simulink model "AUAV_V3_TestSensors_"  (R2015a)
settings: Solver=FixedStepDiscrete  StartTime=0.0  StopTime=10.0  FixedStep=T  RelTol=1e-3
PreLoadFcn:
  | %T = 0.0025;
  | MavlinkBus;
  | mcuInit;
  | % Baro Altitude Computation
  | % =========================
  | basePressure = 98192.64;
  | baseTemp = 288.215;
  | lapseRate = -0.00198122;
  | baseHeight = 0;
values from neighbouring files (symbols this model uses):
  apSampleTime = 0.01    [mcuInit.m]
  latlong_WP = 1    [mcuInit.m]
  mavlink_attitude_t = Simulink.Bus    [MavlinkBusMarcello.m]
  mavlink_gps_raw_int_t = Simulink.Bus    [MavlinkBus.m]    (also in MavlinkBusMarcello.m)
  mavlink_raw_imu_t = Simulink.Bus    [MavlinkBus.m]    (also in MavlinkBusMarcello.m)
  mavlink_scaled_pressure_t = Simulink.Bus    [MavlinkBus.m]    (also in MavlinkBusMarcello.m)
  mavlink_servo_output_raw_t = Simulink.Bus    [MavlinkBusMarcello.m]
  mavlink_sys_status_t = Simulink.Bus    [MavlinkBus.m]    (also in MavlinkBusMarcello.m)
  T = 0.01    [mcuInit.m]
  Xpoints = [0 0]    [mcuInit.m]
  Ypoints = [0 0]    [mcuInit.m]
  Zpoints = [0 0]    [mcuInit.m]
undefined symbols (not defined in the file or in its folder): A0, A14, A15, A2, A3, A4, A5, A6, accBiasRateLimit, B0, bankCommandLimit, barAdjust, baroCutoff, baroCutTemp, cubeAccelGain16405, cubeGyroGain16405, cubeMagGain16405, D0, D11, D7, D8, daLimit, data, daTrimMax, daTrimMin, deLimit, deTrimMax, deTrimMin, drLimit, drTrimMax, drTrimMin, dtLimit, dtTrimMax, dtTrimMin, F2, F3, G0, G13, G15, gaind, GS_location, gyroBiasRateLimit, IC1max, IPStar, ISA_g, Max, maxAcc, MaxDwnPthStar, maxDynPressure, maxEta, mlParamInterface, ms, OC1max, P112, P125, P127, P16, P20, P21, P30 ... (+26)
undefined symbols (not defined in the file): baroOffset, baroScale, barTGain1, barTGain2, barTMean1, barTMean2, bda, bde, bdr, bdt, bICda, bICde, bICdr, bICdt, derivativesConstant, lowRateSensorCutoff, mainSensorCutoff, mda, mde, mdr, mdt, mICda, mICde, mICdr, mICdt, pitotOffset, pitotScale, pitTGain1, pitTGain2, pitTMean1, pitTMean2, powerOffset, powerScale, pressureSensorCutoff, tempOffset, tempScale, vzCutoff, xCutoff, yCutoff
libraries: MCHP_Blockset x150, simulink x84, SLUGS_Library x31, aerolibconvert2 x6, aerolibutil x4, aerolibtransform2 x3, dspmtrx3 x2, aerolibobsolete x2
(part 10 of 20)

== system AUAV_V3_TestSensors_/Sensor_Data_Adapter/Sensor Suite ==
  HIL_flag : Inport
  Raw HIL : Inport  Port=2
  " GPS is Ublox" : Subsystem
  "ADIS16405 Signal Cond " : Subsystem
  Compute CPU Load : Subsystem
  Data Type Conversion{4..7} (4 alike) : DataTypeConversion  OutDataTypeStr=single
  Demux : Demux
  Demux1 : Demux
  Goto4 : Goto  Commented=on  GotoTag=IntDiag
  Goto5 : Goto  Commented=on  GotoTag=charDiag
  If no HIL then Read all the Sensors : Subsystem
  If no HIL then update Air Data : Subsystem
  Logical Operator : Logic  Operator=NOT  AllPortsSameDT=off  OutDataTypeStr=boolean
  Low Pass Filtering,Temperature Compensation and Calibration : Subsystem
  Sensor DSC Diag [updateSensorMcuState.c]1 : MCHP_Blockset/User Functions/C Function Call  ParseFilesChkbx=off  ListFunctions1=Custom Function  Function1=extern void updateSensorDiag(real32_T* u1);  AddHeaderDeclaration=off  Function1Type=when block is updated (default)  Fct1BlockIn=u1[4]  FctReturnBlockOut=off  DataCollected=0  ORDERING=None  SampleTime=.01  MCHP_MASTERLINK=|  PinDigitalInput=[]  PinDigitalOutput=[]  PinAnalogInput=[]
      | AUAV_V3_TestSensors_/Microchip Master
      | AUAV V3 Board
      | Busy Flag on D2 (RA6)
  Switch : Switch  Criteria=u2 ~= 0  SampleTime=0.01
  Switch1 : Switch  Criteria=u2 ~= 0  SampleTime=0.01
  Update the Load and Power Data [updateSensorMcuState.c]1 : MCHP_Blockset/User Functions/C Function Call  ParseFilesChkbx=off  ListFunctions1=Custom Function  Function1=extern void updateLoadData(uint8_T u1, uint16_T u2);  AddHeaderDeclaration=off  Function1Type=when block is updated (default)  FctReturnBlockOut=off  DataCollected=0  ORDERING=None  SampleTime=.01  MCHP_MASTERLINK=|  PinDigitalInput=[]  PinDigitalOutput=[]  PinAnalogInput=[]
      | AUAV_V3_TestSensors_/Microchip Master
      | AUAV V3 Board
      | Busy Flag on D2 (RA6)
  myMux Fun : MATLAB Function  TreatAsAtomicUnit=on
  myMux Fun1 : MATLAB Function  TreatAsAtomicUnit=on
  Omega (rad/s) : Outport
  Accel (m/s^2) : Outport  Port=2
  Mag (mG) : Outport  Port=3
  Baro Alt (m) : Outport  Port=4
  GPS : Outport  Port=5
  wires:
  If no HIL then Read all the Sensors/1(Sensors) -> Switch/3
  Logical Operator/1 -> If no HIL then Read all the Sensors/Enable, [Not_HIL]
  Demux/1 -> "ADIS16405 Signal Cond "/1(Gyro Raw)  "Gyro"
  Demux1/1 -> Low Pass Filtering,Temperature Compensation and Calibration/1(Baro raw)
  Demux1/2 -> Low Pass Filtering,Temperature Compensation and Calibration/2(Pitot raw)
  Demux1/4 -> Low Pass Filtering,Temperature Compensation and Calibration/4(Therm Raw)
  Demux/3 -> "ADIS16405 Signal Cond "/3(Mag Raw)  "Mag"
  Demux1/3 -> Low Pass Filtering,Temperature Compensation and Calibration/3(Power Raw)
  Low Pass Filtering,Temperature Compensation and Calibration/2(Pitot (Pa)) -> myMux Fun/1(u1), [Float1Diag]
  Low Pass Filtering,Temperature Compensation and Calibration/3(Static (Pa)) -> myMux Fun/2(u2)
  myMux Fun/1(y) -> If no HIL then update Air Data/1(AirData)
  Low Pass Filtering,Temperature Compensation and Calibration/4(Temp (0.1 C)) -> myMux Fun/3(u3)
  Compute CPU Load/1(Load (%)) -> Update the Load and Power Data [updateSensorMcuState.c]1/1
  Low Pass Filtering,Temperature Compensation and Calibration/5(Power (V)) -> Update the Load and Power Data [updateSensorMcuState.c]1/2
  Demux/2 -> "ADIS16405 Signal Cond "/2(Accel Raw)  "Accel"
  myMux Fun1/1(y) -> Sensor DSC Diag [updateSensorMcuState.c]1/1
  Data Type Conversion5/1 -> myMux Fun1/1(u1)  "float"
  Data Type Conversion4/1 -> myMux Fun1/2(u2)  "float"
  Data Type Conversion6/1 -> myMux Fun1/3(u3)  "int"
  Data Type Conversion7/1 -> myMux Fun1/4(u4)  "char"
  [Float1Diag] -> Data Type Conversion5/1
  [Float2Diag] -> Data Type Conversion4/1
  [IntDiag] -> Data Type Conversion6/1
  [charDiag] -> Data Type Conversion7/1
  [Not_HIL] -> If no HIL then update Air Data/Enable
  If no HIL then update Air Data/1(Out1) -> [Float2Diag]
  "ADIS16405 Signal Cond "/1(Omega (rad/s)) -> Omega (rad/s)/1
  "ADIS16405 Signal Cond "/2(Accel (m/s^2)) -> Accel (m/s^2)/1
  "ADIS16405 Signal Cond "/3(Mags (mG)) -> Mag (mG)/1
  Raw HIL/1 -> Switch/1
  HIL_flag/1 -> [HIL], Switch/2, Logical Operator/1
  Switch/1 -> Demux/1
  Low Pass Filtering,Temperature Compensation and Calibration/1(Baro Alt (m)) -> Baro Alt (m)/1
  Demux/4 -> Demux1/1
  [Not_HIL] -> Switch1/2
  Switch1/1 -> GPS/1
  " GPS is Ublox"/1(GPS Main) -> Switch1/3
  If no HIL then Read all the Sensors/2(GPS) -> Switch1/1

== system AUAV_V3_TestSensors_/Servo In Out/Convert to Microseconds ==
  PWM : Inport
  Convert to Microseconds : Gain  Gain=0.4
  Data Type Conversion : DataTypeConversion  OutDataTypeStr=uint16
  uS : Outport
  wires:
  Data Type Conversion/1 -> uS/1
  PWM/1 -> Convert to Microseconds/1
  Convert to Microseconds/1 -> Data Type Conversion/1

== system AUAV_V3_TestSensors_/Servo In Out/Convert to Microseconds1 ==
  PWM : Inport
  Convert to Microseconds : Gain  Gain=0.4
  Data Type Conversion : DataTypeConversion  OutDataTypeStr=uint16
  uS : Outport
  wires:
  Data Type Conversion/1 -> uS/1
  PWM/1 -> Convert to Microseconds/1
  Convert to Microseconds/1 -> Data Type Conversion/1

== system AUAV_V3_TestSensors_/Servo In Out/Convert to Microseconds2 ==
  PWM : Inport
  Convert to Microseconds : Gain  Gain=0.4
  Data Type Conversion : DataTypeConversion  OutDataTypeStr=uint16
  uS : Outport
  wires:
  Data Type Conversion/1 -> uS/1
  PWM/1 -> Convert to Microseconds/1
  Convert to Microseconds/1 -> Data Type Conversion/1

== system AUAV_V3_TestSensors_/Servo In Out/Mixing ==
  note: Pitch positif : go down
      | Yaw positive : turn left
  Pitch : Inport
  Roll : Inport  Port=2
  Sum : Sum  Inputs=-+  SaturateOnIntegerOverflow=on  OutDataTypeStr=Inherit: Same as first input
  Sum1 : Sum  SaturateOnIntegerOverflow=on  OutDataTypeStr=Inherit: Same as first input
  Cmd Servo Left : Outport
  Cmd Servo Right : Outport  Port=2
  wires:
  Pitch/1 -> Sum1/1, Sum/1
  Roll/1 -> Sum/2, Sum1/2
  Sum/1 -> Cmd Servo Left/1
  Sum1/1 -> Cmd Servo Right/1

== system AUAV_V3_TestSensors_/Trim Vals [updated 4.28.16]/Bufffer IC ==
  Pilot Console : Inport
  Buffer IC Channel : MATLAB Function  TreatAsAtomicUnit=on
  Buffer IC Channel1 : MATLAB Function  TreatAsAtomicUnit=on
  Buffer IC Channel2 : MATLAB Function  TreatAsAtomicUnit=on
  Buffer IC Channel3 : MATLAB Function  TreatAsAtomicUnit=on
  Demux : Demux
  dT_buf : Outport
  dA_buf : Outport  Port=2
  dR_buf : Outport  Port=3
  dE_buf : Outport  Port=4
  wires:
  Demux/1 -> Buffer IC Channel/1(latest)
  Demux/2 -> Buffer IC Channel1/1(latest)
  Demux/3 -> Buffer IC Channel2/1(latest)
  Demux/4 -> Buffer IC Channel3/1(latest)
  Pilot Console/1 -> Demux/1
  Buffer IC Channel/1(history) -> dT_buf/1
  Buffer IC Channel1/1(history) -> dA_buf/1
  Buffer IC Channel2/1(history) -> dR_buf/1
  Buffer IC Channel3/1(history) -> dE_buf/1

== system AUAV_V3_TestSensors_/Trim Vals [updated 4.28.16]/Control Surface Input ==
  2 sec  tau : Subsystem  mask(Tustin1stOrderLowpassAutoInitialCondition){f=0.1, T=T}
      mask prompts: f "Lowpass Frequency"; T "Sample Time"
      mask help: Takes a 3db rolloff frequency (in Hz, NOT radians/s) and a sample time. Performs a symbolic Tustin conversion and implements in a discrete filter. The initial output of the filter is set by the first sample.
      mask Help: Enter the desired 3db rolloff frequency in Hz and the sample time. Initial conditions are sampled automatically.
      mask Display: fprintf('%.2f Hz lowpass',f)
  2 sec  tau1 : Subsystem  mask(Tustin1stOrderLowpassAutoInitialCondition){f=0.1, T=T}
      mask prompts: f "Lowpass Frequency"; T "Sample Time"
      mask help: Takes a 3db rolloff frequency (in Hz, NOT radians/s) and a sample time. Performs a symbolic Tustin conversion and implements in a discrete filter. The initial output of the filter is set by the first sample.
      mask Help: Enter the desired 3db rolloff frequency in Hz and the sample time. Initial conditions are sampled automatically.
      mask Display: fprintf('%.2f Hz lowpass',f)
  Data Type Conversion1 : DataTypeConversion  OutDataTypeStr=uint16
  Data Type Conversion2 : DataTypeConversion  OutDataTypeStr=single
  Data Type Conversion3 : DataTypeConversion  OutDataTypeStr=single
  Data Type Conversion4 : DataTypeConversion  OutDataTypeStr=uint16
  Input Capture : MCHP_Blockset/Pulse Input//Output/Input Capture  IntPriority=6  Channel="[1     2     3     4     5     6     7     8]"  Channel_OLD="[1  2  3  4  5  6  7  8]"  PIN_IC1=Dynamic Options  PIN_IC1_TXT=D0 / P64 / Pin[72]  PIN_IC2=Dynamic Options  PIN_IC2_TXT=D8 / P72 / Pin[68]  PIN_IC3=Dynamic Options  PIN_IC3_TXT=D11 / P75 / Pin[71]  PIN_IC4=Dynamic Options  PIN_IC4_TXT=A15 / P31 / Pin[67]  PIN_IC5=Dynamic Options  PIN_IC5_TXT=A5 / P21 / Pin[61]  PIN_IC6=Dynamic Options  PIN_IC6_TXT=A14 / P30 / Pin[66]  PIN_IC7=Dynamic Options  PIN_IC7_TXT=A4 / P20 / Pin[60]  PIN_IC8=Dynamic Options  PIN_IC8_TXT=A0 / P16 / Pin[17]  PIN_IC9=Dynamic Options  PIN_IC9_TXT=A0 / P16 / Pin[17]  PIN_IC10=Dynamic Options  PIN_IC10_TXT=A0 / P16 / Pin[17]  PIN_IC11=Dynamic Options  PIN_IC11_TXT=A0 / P16 / Pin[17]  PIN_IC12=Dynamic Options  PIN_IC12_TXT=A0 / P16 / Pin[17]  PIN_IC13=Dynamic Options  PIN_IC13_TXT=A0 / P16 / Pin[17]  PIN_IC14=Dynamic Options  PIN_IC14_TXT=A0 / P16 / Pin[17]  PIN_IC15=Dynamic Options  PIN_IC15_TXT=A0 / P16 / Pin[17]  PIN_IC16=Dynamic Options  PIN_IC16_TXT=A0 / P16 / Pin[17]  Channel_UP_Down_Periode="[1     1     1     1     1     1     1     1]"  MaxChannel="[0.003   0.003   0.003   0.003   0.003   0.003   0.003   0.003]"  SafeMarge="[0     0     0     0     0     0     0     0]"  MaxChannelValue="2.^[ 14.680  14.680  14.680  14.680  14.680  14.680  14.680  14.680]  =>  [26249  26249  26249  26249  26249  26249  26249  26249]"  ICxmax="[26249  26249  26249  26249  26249  26249  26249  26249]"  Timer="[1  1  1  1  1  1  1  1]"  ChangeDetected="[0     0     0     0     0     0     0     0]"  ChangeDetectedPortRef=3  SampleTime=.01  Status=OK  MCHP_PORT={Input Capture 1}{IC1}6:0:P64;{Input Capture 2}{IC2}6:0:P72;{Input Capture 3}{IC3}6:0:P75;{Input Capture 4}{IC4}6:0:P31;{Input Capture 5}{IC5}6:0:P21;{Input Capture 6}{IC6}6:0:P30;{Input Capture 7}{IC7}6:0:P20;{Input Capture 8}{IC8}6:0:P16;  MCHP_TIMER_REQUEST="{Input Capture 1}{IC1}6:0:1:0:[1  2  3  4  5]:210000;{Input Capture 1}{IC1}6:0:1:0:[1  2  3  4  5]:210000;{Input Capture 1}{IC1}6:0:1:0:[1  2  3  4  5]:210000;{Input Capture 1}{IC1}6:0:1:0:[1  2  3  4  5]:210000;{Input Capture 1}{IC1}6:0:1:0:[1  2  3  4  5]:210000;{Input Capture 1}{IC1}6:0:1:0:[1  2  3  4  5]:210000;{Input Capture 1}{IC1}6:0:1:0:[1  2  3  4  5]:210000;{Input Capture 1}{IC1}6:0:1:0:[1  2  3  4  5]:210000;"  MCHP_TIMER_RESULT=[1 26249.000000000011 ;1 26249.000000000011 ;1 26249.000000000011 ;1 26249.000000000011 ;1 26249.000000000011 ;1 26249.000000000011 ;1 26249.000000000011 ;1 26249.000000000011 ]  MCHP_MASTERLINK=|
      | AUAV_V3_TestSensors/Microchip Master
      | AUAV V3 Board
      | Busy Flag on D2 (RA6)
  Update Control Surface DATA : DataStoreWrite  DialogController=Simulink.DDGSource  DataStoreName=mlPilotConsoleData  DataStoreElements=mlPilotConsoleData.chan1_raw#mlPilotConsoleData.chan2_raw#mlPilotConsoleData.chan3_raw#mlPilotConsoleData.chan4_raw#mlPilotConsoleData.chan5_raw#mlPilotConsoleData.chan6_raw#mlPilotConsoleData.chan7_raw#mlPilotConsoleData.chan8_raw
  myMux Fun1 : MATLAB Function  TreatAsAtomicUnit=on
  myMux Fun5 : MATLAB Function  TreatAsAtomicUnit=on
  Pilot Console : Outport
  Voltage/Current Sensor : Outport  Port=2
  wires:
  Input Capture/7 -> Data Type Conversion3/1, Update Control Surface DATA/7
  myMux Fun1/1(y) -> Voltage/Current Sensor/1
  Input Capture/6 -> Update Control Surface DATA/6, Data Type Conversion2/1
  2 sec  tau/1(Out1) -> Data Type Conversion1/1
  2 sec  tau1/1(Out1) -> Data Type Conversion4/1
  Data Type Conversion1/1 -> myMux Fun1/1(u1)
  Data Type Conversion4/1 -> myMux Fun1/2(u2)
  Data Type Conversion2/1 -> 2 sec  tau/1(In1)
  Data Type Conversion3/1 -> 2 sec  tau1/1(In1)
  Input Capture/1 -> myMux Fun5/1(u1), Update Control Surface DATA/1
  Input Capture/4 -> myMux Fun5/4(u4), Update Control Surface DATA/4
  Input Capture/5 -> myMux Fun5/5(u5), Update Control Surface DATA/5
  Input Capture/2 -> myMux Fun5/2(u2), Update Control Surface DATA/2
  Input Capture/3 -> myMux Fun5/3(u3), Update Control Surface DATA/3
  myMux Fun5/1(y) -> Pilot Console/1
  Input Capture/8 -> Update Control Surface DATA/8

== system AUAV_V3_TestSensors_/Trim Vals [updated 4.28.16]/Convert to Microseconds  ==
  IC : Inport
  Convert to Microseconds : Gain  Gain=0.2
  Data Type Conversion : DataTypeConversion  OutDataTypeStr=uint16
  uS : Outport
  wires:
  Convert to Microseconds/1 -> Data Type Conversion/1
  IC/1 -> Convert to Microseconds/1
  Data Type Conversion/1 -> uS/1

== system AUAV_V3_TestSensors_/Trim Vals [updated 4.28.16]/Detect Transition High to Low ==
  Switch : Inport
  IC1 : InitialCondition  Value=0
  Logical Operator : Logic  Operator=NOT  AllPortsSameDT=off  OutDataTypeStr=boolean
  Subsystem : Subsystem
  Transition : Outport
  wires:
  Switch/1 -> Logical Operator/1
  IC1/1 -> Subsystem/1(WP Fly)
  Logical Operator/1 -> IC1/1
  Subsystem/1(Just Enab) -> Transition/1

== system AUAV_V3_TestSensors_/Trim Vals [updated 4.28.16]/Grab I.C. ==
  dT_buf : Inport
  dA_buf : Inport  Port=2
  dR_buf : Inport  Port=3
  dE_buf : Inport  Port=4
  Enable : EnablePort
  2 : MCHP_Blockset/User Functions/C Function Call  ParseFilesChkbx=off  ListFunctions1=Custom Function  Function1=extern uint16_T meanFilter5(uint16_T* u1);  AddHeaderDeclaration=off  Function1Type=when block is updated (default)  FctReturnBlockOut=on  Fct1BlockOut=y1  DataCollected=0  ORDERING=None  SampleTime=-1  MCHP_MASTERLINK=|  PinDigitalInput=[]  PinDigitalOutput=[]  PinAnalogInput=[]
      | AUAV_V3_TestSensors_/Microchip Master
      | AUAV V3 Board
      | Busy Flag on D2 (RA6)
  3 : MCHP_Blockset/User Functions/C Function Call  ParseFilesChkbx=off  ListFunctions1=Custom Function  Function1=extern uint16_T meanFilter5(uint16_T* u1);  AddHeaderDeclaration=off  Function1Type=when block is updated (default)  FctReturnBlockOut=on  Fct1BlockOut=y1  DataCollected=0  ORDERING=None  SampleTime=-1  MCHP_MASTERLINK=|  PinDigitalInput=[]  PinDigitalOutput=[]  PinAnalogInput=[]
      | AUAV_V3_TestSensors_/Microchip Master
      | AUAV V3 Board
      | Busy Flag on D2 (RA6)
  4 : MCHP_Blockset/User Functions/C Function Call  ParseFilesChkbx=off  ListFunctions1=Custom Function  Function1=extern uint16_T meanFilter5(uint16_T* u1);  AddHeaderDeclaration=off  Function1Type=when block is updated (default)  FctReturnBlockOut=on  Fct1BlockOut=y1  DataCollected=0  ORDERING=None  SampleTime=-1  MCHP_MASTERLINK=|  PinDigitalInput=[]  PinDigitalOutput=[]  PinAnalogInput=[]
      | AUAV_V3_TestSensors_/Microchip Master
      | AUAV V3 Board
      | Busy Flag on D2 (RA6)
  Choose the Median navSupport.c [updated 4.28.16] : MCHP_Blockset/User Functions/C Function Call  ParseFilesChkbx=off  ListFunctions1=Custom Function  Function1=extern uint16_T meanFilter5(uint16_T* u1);  AddHeaderDeclaration=off  Function1Type=when block is updated (default)  FctReturnBlockOut=on  Fct1BlockOut=y1  DataCollected=0  ORDERING=None  SampleTime=-1  MCHP_MASTERLINK=|  PinDigitalInput=[]  PinDigitalOutput=[]  PinAnalogInput=[]
      | AUAV_V3_TestSensors_/Microchip Master
      | AUAV V3 Board
      | Busy Flag on D2 (RA6)
  "Convert to Microseconds " : Subsystem
  Convert to Microseconds 1 : Subsystem
  Convert to Microseconds 2 : Subsystem
  Convert to Microseconds 3 : Subsystem
  Convert to Rad : Subsystem  mask{slopem=mICdt, interceptb=bICdt}
      mask prompts: slopem "Slope"; interceptb "Intercept"
  Convert to Rad1 : Subsystem  mask{slopem=mICda, interceptb=bICda}
      mask prompts: slopem "Slope"; interceptb "Intercept"
  Convert to Rad2 : Subsystem  mask{slopem=mICdr, interceptb=bICdr}
      mask prompts: slopem "Slope"; interceptb "Intercept"
  Convert to Rad3 : Subsystem  mask{slopem=mICde, interceptb=bICde}
      mask prompts: slopem "Slope"; interceptb "Intercept"
  "[-2  2] deg" : Saturate  UpperLimit=daTrimMax  LowerLimit=daTrimMin
  "[-2  2] deg " : Saturate  UpperLimit=drTrimMax  LowerLimit=drTrimMin
  "[-2  2] deg  " : Saturate  UpperLimit=deTrimMax  LowerLimit=deTrimMin
  "[0.55 0.68]" : Saturate  UpperLimit=dtTrimMax  LowerLimit=dtTrimMin
  dA : Constant  OutDataTypeStr=uint8
  dE : Constant  Value=3  OutDataTypeStr=uint8
  dR : Constant  Value=2  OutDataTypeStr=uint8
  dT : Constant  Value=0  OutDataTypeStr=uint8
  update dA Trim updateControlMcu.c : MCHP_Blockset/User Functions/C Function Call  ParseFilesChkbx=off  ListFunctions1=Custom Function  Function1=extern void updatePWMTrim(uint16_T* u1, uint8_T* u2);  AddHeaderDeclaration=off  Function1Type=when block is updated (default)  FctReturnBlockOut=on  DataCollected=0  ORDERING=None  SampleTime=-1  MCHP_MASTERLINK=|  PinDigitalInput=[]  PinDigitalOutput=[]  PinAnalogInput=[]
      | AUAV_V3_TestSensors_/Microchip Master
      | AUAV V3 Board
      | Busy Flag on D2 (RA6)
  update dE Trim updateControlMcu.c : MCHP_Blockset/User Functions/C Function Call  ParseFilesChkbx=off  ListFunctions1=Custom Function  Function1=extern void updatePWMTrim(uint16_T* u1, uint8_T* u2);  AddHeaderDeclaration=off  Function1Type=when block is updated (default)  FctReturnBlockOut=on  DataCollected=0  ORDERING=None  SampleTime=-1  MCHP_MASTERLINK=|  PinDigitalInput=[]  PinDigitalOutput=[]  PinAnalogInput=[]
      | AUAV_V3_TestSensors_/Microchip Master
      | AUAV V3 Board
      | Busy Flag on D2 (RA6)
  update dR Trim updateControlMcu.c : MCHP_Blockset/User Functions/C Function Call  ParseFilesChkbx=off  ListFunctions1=Custom Function  Function1=extern void updatePWMTrim(uint16_T* u1, uint8_T* u2);  AddHeaderDeclaration=off  Function1Type=when block is updated (default)  FctReturnBlockOut=on  DataCollected=0  ORDERING=None  SampleTime=-1  MCHP_MASTERLINK=|  PinDigitalInput=[]  PinDigitalOutput=[]  PinAnalogInput=[]
      | AUAV_V3_TestSensors_/Microchip Master
      | AUAV V3 Board
      | Busy Flag on D2 (RA6)
  update dT Trim updateControlMcu.c [updated 4.28.16] : MCHP_Blockset/User Functions/C Function Call  ParseFilesChkbx=off  ListFunctions1=Custom Function  Function1=extern void updatePWMTrim(uint16_T* u1, uint8_T* u2);  AddHeaderDeclaration=off  Function1Type=when block is updated (default)  FctReturnBlockOut=on  DataCollected=0  ORDERING=None  SampleTime=-1  MCHP_MASTERLINK=|  PinDigitalInput=[]  PinDigitalOutput=[]  PinAnalogInput=[]
      | AUAV_V3_TestSensors_/Microchip Master
      | AUAV V3 Board
      | Busy Flag on D2 (RA6)
  dT_trim (abs) : Outport
  dA_trim (rad) : Outport  Port=2
  dR_trim (rad) : Outport  Port=3
  dE_trim (rad) : Outport  Port=4
  wires:
  Convert to Rad/1(Angle (rad)) -> dT_trim (abs)/1
  Convert to Rad2/1(Angle (rad)) -> dR_trim (rad)/1
  Convert to Rad3/1(Angle (rad)) -> dE_trim (rad)/1
  Choose the Median navSupport.c [updated 4.28.16]/1 -> "[0.55 0.68]"/1
  2/1 -> "[-2  2] deg"/1
  3/1 -> "[-2  2] deg "/1
  4/1 -> "[-2  2] deg  "/1
  dT_buf/1 -> Choose the Median navSupport.c [updated 4.28.16]/1
  dA_buf/1 -> 2/1
  dR_buf/1 -> 3/1
  dR/1 -> update dR Trim updateControlMcu.c/2
  dE/1 -> update dE Trim updateControlMcu.c/2
  dT/1 -> update dT Trim updateControlMcu.c [updated 4.28.16]/2
  dA/1 -> update dA Trim updateControlMcu.c/2
  "[0.55 0.68]"/1 -> Convert to Rad/1(IC), "Convert to Microseconds "/1(IC)
  "[-2  2] deg"/1 -> Convert to Rad1/1(IC), Convert to Microseconds 1/1(IC)
  "[-2  2] deg "/1 -> Convert to Rad2/1(IC), Convert to Microseconds 2/1(IC)
  "[-2  2] deg  "/1 -> Convert to Rad3/1(IC), Convert to Microseconds 3/1(IC)
  Convert to Rad1/1(Angle (rad)) -> dA_trim (rad)/1
  "Convert to Microseconds "/1(uS) -> update dT Trim updateControlMcu.c [updated 4.28.16]/1
  Convert to Microseconds 1/1(uS) -> update dA Trim updateControlMcu.c/1
  Convert to Microseconds 2/1(uS) -> update dR Trim updateControlMcu.c/1
  Convert to Microseconds 3/1(uS) -> update dE Trim updateControlMcu.c/1
  dE_buf/1 -> 4/1

== system AUAV_V3_TestSensors_/Trim Vals [updated 4.28.16]/Mean Filter the Transition ==
  Failsafe : Inport
  Buffer Failsafe Channel : MATLAB Function  TreatAsAtomicUnit=on
  Choose the Median [navSupport.c] [updated 5.1.16] : MCHP_Blockset/User Functions/C Function Call  ParseFilesChkbx=off  ListFunctions1=Custom Function  Function1=extern uint16_T meanFilter5(uint8_T *u1);  AddHeaderDeclaration=on  Function1Type=when block is updated (default)  Fct1BlockIn=u1  FctReturnBlockOut=on  DataCollected=0  ORDERING=None  SampleTime=-1  MCHP_MASTERLINK=|  PinDigitalInput=[]  PinDigitalOutput=[]  PinAnalogInput=[]
      | AUAV_V3_TestSensors_/Microchip Master
      | AUAV V3 Board
      | Busy Flag on D2 (RA6)
  Data Type Conversion : DataTypeConversion  OutDataTypeStr=uint16
  Data Type Conversion1 : DataTypeConversion  OutDataTypeStr=uint8
  filtered : Outport
  wires:
  Choose the Median [navSupport.c] [updated 5.1.16]/1 -> filtered/1
  Data Type Conversion/1 -> Buffer Failsafe Channel/1(latest)
  Failsafe/1 -> Data Type Conversion/1
  Data Type Conversion1/1 -> Choose the Median [navSupport.c] [updated 5.1.16]/1
  Buffer Failsafe Channel/1(history) -> Data Type Conversion1/1

== system AUAV_V3_TestSensors_/Update PWM Commands and Send Telemetry [updated 4.27.16]/Convert to Microseconds ==
  PWM : Inport
  Convert to Microseconds : Gain  Gain=0.2
  Data Type Conversion : DataTypeConversion  OutDataTypeStr=uint16
  uS : Outport
  wires:
  Data Type Conversion/1 -> uS/1
  PWM/1 -> Convert to Microseconds/1
  Convert to Microseconds/1 -> Data Type Conversion/1

== system AUAV_V3_TestSensors_/Update PWM Commands and Send Telemetry [updated 4.27.16]/Generate PWM Signals Based on the Control Type ==
  note: Navigation Modes:
      | 2 -> PT
      | 3 -> Waypoint
      | 4 -> Mid Level
      | 8-> Sel PT
      | 9-> ISR
      | 10 -> Line Patrol
  PWM(rad) : Inport
  Pilot Console (IC) : Inport  Port=2
  isManual? : Inport  Port=3
  Nav Mode : Inport  Port=4
  Data Type Conversion : DataTypeConversion  OutDataTypeStr=uint16
  Data Type Conversion1 : DataTypeConversion  OutDataTypeStr=uint8
  If : If  NumInputs=2  IfExpression=u2 == 1  ElseIfExpressions=((u1 == 3) | (u1 == 4) | (u1 == 9) | (u1 == 10)), u1 == 2, u1 == 8  ShowElse=off  SampleTime=.01
  If  Control Type Is Manual : Subsystem  TreatAsAtomicUnit=on
  If  Control Type Is Passthrough : Subsystem  TreatAsAtomicUnit=on
  If  Control Type Is Selective Passthrough : Subsystem  TreatAsAtomicUnit=on
  "If  Control Type Is Wp, ISR, LP or  Mid Lvl Cmds" : Subsystem  TreatAsAtomicUnit=on
  Merge : Merge  Inputs=4
  PWM : Outport
  wires:
  If/1 -> If  Control Type Is Manual/Action
  If/2 -> "If  Control Type Is Wp, ISR, LP or  Mid Lvl Cmds"/Action
  If/3 -> If  Control Type Is Passthrough/Action
  If/4 -> If  Control Type Is Selective Passthrough/Action
  If  Control Type Is Manual/1(PWM) -> Merge/1
  "If  Control Type Is Wp, ISR, LP or  Mid Lvl Cmds"/1(PWM (abs)) -> Merge/2
  If  Control Type Is Passthrough/1(PWM (abs)) -> Merge/3
  If  Control Type Is Selective Passthrough/1(PWM) -> Merge/4
  PWM(rad)/1 -> "If  Control Type Is Wp, ISR, LP or  Mid Lvl Cmds"/1(PWM(rad)), If  Control Type Is Selective Passthrough/1(PWM(rad))
  Pilot Console (IC)/1 -> If  Control Type Is Manual/1(Pilot (IC)), If  Control Type Is Passthrough/1(Pilot (IC)), If  Control Type Is Selective Passthrough/2(Pilot (IC))
  Merge/1 -> Data Type Conversion/1
  Data Type Conversion/1 -> PWM/1
  isManual?/1 -> If/2
  Nav Mode/1 -> Data Type Conversion1/1
  Data Type Conversion1/1 -> If/1

== system AUAV_V3_TestSensors_/Update PWM Commands and Send Telemetry [updated 4.27.16]/Send_Cmd_HIL ==
  Enable : EnablePort
  COMP_ID : Constant  OutDataTypeStr=uint8
  Get Raw Commands : DataStoreRead  DialogController=Simulink.DDGSource  DataStoreName=mlPwmCommands  DataStoreElements=mlPwmCommands
  Get time5 : DataStoreRead  DataStoreName=time_since_boot_usec  DataStoreElements=time_since_boot_usec
  PackRawServo : MCHP_Blockset/User Functions/C Function Call  ParseFilesChkbx=on  ListFunctions1=Custom Function  Function1=uint16_t HIL_PackRawServo(uint8_t system_id, uint8_t component_id, mavlink_servo_output_raw_t mlPwmCommands ,uint32_t time_usec)  AddHeaderDeclaration=on  Function1Type=when block is updated (default)  Fct1BlockIn="system_id  , component_id  , mlPwmCommands  , time_usec"  FctReturnBlockOut=on  DataCollected="s.chksm=reshape({ '638503-Feb-2015 20:58:10','251913-Sep-2016 12:15:14','1628414-Sep-2016 10:06:29','3754120-Sep-2016 10:12:03','360317-Jun-2016 15:34:16','7114620-Sep-2016 10:38:54','954931-Aug-2016 15:03:40','295520-Sep-2016 10:30:42','268124-Jun-2016 00:23:34','556017-Jun-2016 15:34:16','963217-Jun-2016 15:34:16','1086024-Jun-2016 00:23:34','372414-Sep-2016 14:01:55','998814-Sep-2016 11:55:45','509015-Sep-2016 09:12:19'},1,15);s.File1=reshape({ '  void  newCircBuffer(CBRef cB)','  void  freeCircBuffer(CBRef* cB)','  void  freeCircBuffer(CBRef* cB)',' unsigned int  getLength(CBRef cB)','  int  readHead(CBRef cB)','  int  readTail(CBRef cB)',' unsigned char  peak(CBRef cB)',' unsigned char  readFront(CBRef cB)',' unsigned char  writeBack(CBRef cB, unsigned char data)','  void  makeEmpty(CBRef cB)','  void  printCircBuf(CBRef cB)'},1,11);s.File2=reshape({ '  void  uartBufferInit(void)','  void  __attribute__((__interrupt__, no_auto_psv)) _U4RXInterrupt(void)','  void  getGPSRawData(unsigned char* gpsBuffer)',' unsigned char  isGPSNovatel(void)'},1,4);s.File3=reshape({ '  char  hex2char(char halfhex)','  float  degMinToDeg(unsigned char degrees, float minutes)',' unsigned char  gpsUbloxSeparate(unsigned char* outStream)','  void  gpsUbloxParse(void)','  void  getGpsUbloxMainData(float* data)','  char  gpSmbl(char symbl)',' unsigned char  myTokenizer(char* stringToTokenize, char token, char * returnToken)','  void  parseRMC(unsigned char* stream)','  void  parseGGA(unsigned char* stream)',' unsigned char  getChecksum(unsigned char* sentence, unsigned char size)','  void  gpsDebugMsg(unsigned char buf)'},1,11);s.File4=reshape({ '  void  uartMavlinkBufferInit(void)','  void __attribute__((__interrupt__,__auto_psv__)) _U1RXInterrupt(void)','  uint8_t  isFinite(float s)','  void  InitParameterInterface(void)','  void  protDecodeMavlink(void)','  uint16_t  MissionInterfaceResponse(uint8_t system_id, uint8_t component_id)','  uint16_t  ParameterInterfaceResponse(uint8_t system_id, uint8_t component_id)','  uint16_t  PackHeartBeat(uint8_t system_id, uint8_t component_id)','  uint16_t  PackTextMsg(uint8_t system_id, uint8_t component_id, unsigned char buf)','  uint16_t  PackRawIMU(uint8_t system_id, uint8_t component_id, mavlink_raw_imu_t mlRawIMUData ,uint32_t time_usec)','  uint16_t  PackGpsRawInt(uint8_t system_id, uint8_t component_id, mavlink_gps_raw_int_t mlRawGpsDataInt ,uint32_t time_usec)','  uint16_t  PackScaledPressure(uint8_t system_id, uint8_t component_id, mavlink_scaled_pressure_t mlAirData ,uint32_t time_usec)','  uint16_t  PackSysStatus(uint8_t system_id, uint8_t component_id, mavlink_sys_status_t mlSysStatus)','  uint16_t  PackRawServo(uint8_t system_id, uint8_t component_id, mavlink_servo_output_raw_t mlPwmCommands ,uint32_t time_usec)','  uint16_t  HIL_PackRawServo(uint8_t system_id, uint8_t component_id, mavlink_servo_output_raw_t mlPwmCommands ,uint32_t time_usec)','  uint16_t  PackRawRC(uint8_t system_id, uint8_t component_id, mavlink_rc_channels_raw_t mlRC_Commands ,uint32_t time_usec)','  uint16_t  PackVFR_HUD(uint8_t system_id, uint8_t component_id, mavlink_vfr_hud_t mlVfr_hud ,uint32_t time_usec)','  char  sendQGCDebugMessage(const char * dbgMessage, char severity, unsigned char* bytesToAdd, char positionStart)','  void  TxN_Data_OverU1(uint16_t N)','  void  TxN_Data_OverU4(uint16_t N)'},1,20);s.File5=reshape({ '  float  myAtan2(float num, float denom)','  float  myPow(float x, float toTheN)','  float  mySqrt(float x)','  float  myAbs(float x)','  float  myAtan(float x)','  float  myAsin(float x)','  float  mySin(float x)','  float  myCos(float x)','  float  myTan(float x)','  float  myAcos(float x)','  float  myExp(float x)','  void  hugeDelay(void)','  void  smallDelay(void)','  void  tinyDelay(void)','  void  printToUart2(const char *fmt, ...)'},1,15);s.File6=reshape({ '  void  sendTelemetryMavlink(unsigned char* dataOut)','  void  uart2Init(void)','  void  gsRead(unsigned char* gsChunk)','  void  prepareTelemetryMavlink(unsigned char* dataOut)','  void  prepareTelemetryMavlink(unsigned char* dataOut)','  void  sendTelemetryMavlink(unsigned char* dataOut)','  void  copyBufferToDMA1(unsigned char size)','  void  send2GS(unsigned char* protData)','  uint8_t  clearWaypointsFrom(uint8_t startingWp)','  void  addMessageToSpiOut(mavlink_message_t* msg)'},1,10);s.File7={ '  void  populateParameterInterface(void)'};s.File8={ '  void  mavlinkInit(void)'};s.File9=reshape({ '  void  updatePWM(unsigned short * PWMData)','  void  updatePWMTrim(unsigned short PWMData, unsigned char channel)','  void  updateLoad(uint8_t mcuLoad)','  void  updateEuler(float* newEuler)','  void  updatePQR(float* newPQR)',' unsigned char  getHilOnOff(void)','  uint8_t  getLightsOnOff(void)','  uint8_t  getLightsDayNight(void)','  void  updateVISensor(uint16_t* data)','  void  updatePTZ(int16_t* ptz)'},1,10);s.File10=reshape({ '  void  updateRawADCData(int16_t* adcData)','  void  updateAirData(float* airData)','  void  updateLoadData(uint8_t load, uint16_t mvPower)','  void  updateAttitude(float * attitudeData)','  void  getGSLocation(float* altLatLon)','  void  updateTimeStamp(uint32_t timeSt)','  void  updatePosition(float * posData)','  void  updatePilotConsole(uint16_t * pilData)','  void  updateDiagnosticFl(float* diagFl)','  void  updateDiagnosticSh(int16_t* diagSh)','  void  updateBias(float * biasData)','  void  updateSensorData(float* sens)','  uint8_t  isFixValid(void)','  void  updateSensorDiag(float* diag)'},1,14);s.File11=reshape({ '  void  gpsInit(void)','  void  gpsParse(uint8_t* dataStream)','  void  updateStatus(uint8_t* completeMessage)','  void  updatePositionData(uint8_t* completeMessage)','  void  updateVelocityData(uint8_t* completeMessage)','  void  updateTimeData(uint8_t* completeMessage)','  void  getGpsMainData(float* data)','  uint32_t  CRC32Value(int32_t i)','  uint32_t  CalculateBlockCRC32(uint32_t ulCount, uint8_t *ucBuffer)','  uint16_t  charsToUint16(uint8_t* data)','  uint32_t  charsToUint32(uint8_t* data)','  float  charsToFloat(uint8_t* data)','  double  charsToDouble(uint8_t* data)'},1,13);s.File12=reshape({ '  void  getMidLevelCommands(float* commands)',' unsigned char  isApManual(uint16_t failsafe)','  float  getParamIdx(unsigned char idx)','  void  getRangeOfParams(uint8_t startIdx, uint8_t endIdx, float* parameters)','  float  getDynamic(void)','  void  getAttitude(float* attitude)','  void  getXYZ(float* xyz)','  void  getVned(float* xyz)','  uint8_t  getMaxWp(void)',' unsigned char  isWpFly(void)',' unsigned char  isPassthrough(void)','  void  setDiagnosticFloat(float * flValues)','  void  setDiagnosticShort(int16_t* shValues)','  void  getWP(unsigned char idx, float* WPpos)','  void  setLogFloat1(float * flValues)','  void  setLogFloat2(float * flValues)',' unsigned char  getApControlType(void)',' unsigned char  getPassValues(uint8_t* pasVals)','  void  setCurrentCommands(float airSpeed)','  void  getCurrentGPSPos(float* latLonAlt)','  void  setNavLong(float* values)','  void  setNavLat(float* values)','  void  setNavNav(float* values)','  void  getAccels(float * accels)','  void  getAccBias(float * bias)','  void  getRTB(uint8_t* rtb)','  void  getMobileLocation(float* loc)','  uint8_t  getNavMode(void)','  void  getISRLocation(float* loc)','  uint8_t  getISRCameraOption1(void)',' unsigned short  meanFilter5(unsigned short * values)','  uint8_t  justEnabled(uint8_t enableValue, uint8_t index)',' unsigned char  quickSort(unsigned short *arr, char elements)'},1,33);s.File13=reshape({ '  void  hilRead(unsigned char* hilChunk)','  void  hil_getRawRead(short * rawData)','  void  hil_getVned(float* vned)','  void  hil_getEuler(float* euler)','  void  hil_getRates(float* pqr)','  void  hil_getXYZ(float* xyz)',' unsigned int  hil_getTs(void)','  void  protDecodeHil(uint8_t* dataIn)'},1,8);s.File14=reshape({ '  void  cubeInit(void)','  void  getCubeData(short * cubeData)','  void  updateCubeData(void)','  int16_t  averageData(int16_t* theData, uint8_t count)',' unsigned short  write2Cube(unsigned short data2Send)','  short  convert14BitToShort(short wordData)','  short  convert12BitToShort(short wordData)',' unsigned char  isCube16405(void)'},1,8);s.File15=reshape({ '  void  uartMavlinkBufferInit(void)','  uint16_t  PackHeartBeat(uint8_t system_id, uint8_t component_id)','  uint16_t  PackRawServo(uint8_t system_id, uint8_t component_id, mavlink_servo_output_raw_t mlPwmCommands ,uint32_t time_usec)','  uint16_t  HIL_PackRawServo(uint8_t system_id, uint8_t component_id, mavlink_servo_output_raw_t mlPwmCommands ,uint32_t time_usec)','  uint16_t  PackRawRC(uint8_t system_id, uint8_t component_id, mavlink_rc_channels_raw_t mlRC_Commands, uint32_t time_usec)','  uint16_t  PackVFR_HUD(uint8_t system_id, uint8_t component_id, mavlink_vfr_hud_t mlVfr_hud, uint32_t time_usec)','  uint16_t  PackRawIMU(uint8_t system_id, uint8_t component_id, mavlink_raw_imu_t mlRawIMUData ,uint32_t time_usec)','  char  sendQGCDebugMessage(const char * dbgMessage, char severity, unsigned char* bytesToAdd, char positionStart)','  uint16_t  PackGpsRawInt(uint8_t system_id, uint8_t component_id, mavlink_gps_raw_int_t mlRawGpsDataInt, uint32_t time_usec)','  uint16_t  PackScaledPressure(uint8_t system_id, uint8_t component_id, mavlink_scaled_pressure_t mlAirData, uint32_t time_usec)','  uint16_t  PackSysStatus(uint8_t system_id, uint8_t component_id, mavlink_sys_status_t mlSysStatus)'},1,11);"  ORDERING=None  SampleTime=-1  MCHP_MASTERLINK=|  PinDigitalInput=[]  PinDigitalOutput=[]  PinAnalogInput=[]
      | AUAV_V3_TestSensors_/Microchip Master
      | AUAV V3 Board
      | Busy Flag on D2 (RA6)
  SYS_ID : Constant  Value=101  OutDataTypeStr=uint8
  TX_N_Data9 : MCHP_Blockset/User Functions/C Function Call  ParseFilesChkbx=on  ListFunctions1=Custom Function  Function1=void TxN_Data_OverU4(uint16_t N)  AddHeaderDeclaration=on  Function1Type=when block is updated (default)  Fct1BlockIn=N  FctReturnBlockOut=on  DataCollected="s.chksm=reshape({ '638503-Feb-2015 20:58:10','251913-Sep-2016 12:15:14','1628414-Sep-2016 10:06:29','3754120-Sep-2016 10:12:03','360317-Jun-2016 15:34:16','7114620-Sep-2016 10:38:54','954931-Aug-2016 15:03:40','295520-Sep-2016 10:30:42','268124-Jun-2016 00:23:34','556017-Jun-2016 15:34:16','963217-Jun-2016 15:34:16','1086024-Jun-2016 00:23:34','372414-Sep-2016 14:01:55','998814-Sep-2016 11:55:45','509015-Sep-2016 09:12:19'},1,15);s.File1=reshape({ '  void  newCircBuffer(CBRef cB)','  void  freeCircBuffer(CBRef* cB)','  void  freeCircBuffer(CBRef* cB)',' unsigned int  getLength(CBRef cB)','  int  readHead(CBRef cB)','  int  readTail(CBRef cB)',' unsigned char  peak(CBRef cB)',' unsigned char  readFront(CBRef cB)',' unsigned char  writeBack(CBRef cB, unsigned char data)','  void  makeEmpty(CBRef cB)','  void  printCircBuf(CBRef cB)'},1,11);s.File2=reshape({ '  void  uartBufferInit(void)','  void  __attribute__((__interrupt__, no_auto_psv)) _U4RXInterrupt(void)','  void  getGPSRawData(unsigned char* gpsBuffer)',' unsigned char  isGPSNovatel(void)'},1,4);s.File3=reshape({ '  char  hex2char(char halfhex)','  float  degMinToDeg(unsigned char degrees, float minutes)',' unsigned char  gpsUbloxSeparate(unsigned char* outStream)','  void  gpsUbloxParse(void)','  void  getGpsUbloxMainData(float* data)','  char  gpSmbl(char symbl)',' unsigned char  myTokenizer(char* stringToTokenize, char token, char * returnToken)','  void  parseRMC(unsigned char* stream)','  void  parseGGA(unsigned char* stream)',' unsigned char  getChecksum(unsigned char* sentence, unsigned char size)','  void  gpsDebugMsg(unsigned char buf)'},1,11);s.File4=reshape({ '  void  uartMavlinkBufferInit(void)','  void __attribute__((__interrupt__,__auto_psv__)) _U1RXInterrupt(void)','  uint8_t  isFinite(float s)','  void  InitParameterInterface(void)','  void  protDecodeMavlink(void)','  uint16_t  MissionInterfaceResponse(uint8_t system_id, uint8_t component_id)','  uint16_t  ParameterInterfaceResponse(uint8_t system_id, uint8_t component_id)','  uint16_t  PackHeartBeat(uint8_t system_id, uint8_t component_id)','  uint16_t  PackTextMsg(uint8_t system_id, uint8_t component_id, unsigned char buf)','  uint16_t  PackRawIMU(uint8_t system_id, uint8_t component_id, mavlink_raw_imu_t mlRawIMUData ,uint32_t time_usec)','  uint16_t  PackGpsRawInt(uint8_t system_id, uint8_t component_id, mavlink_gps_raw_int_t mlRawGpsDataInt ,uint32_t time_usec)','  uint16_t  PackScaledPressure(uint8_t system_id, uint8_t component_id, mavlink_scaled_pressure_t mlAirData ,uint32_t time_usec)','  uint16_t  PackSysStatus(uint8_t system_id, uint8_t component_id, mavlink_sys_status_t mlSysStatus)','  uint16_t  PackRawServo(uint8_t system_id, uint8_t component_id, mavlink_servo_output_raw_t mlPwmCommands ,uint32_t time_usec)','  uint16_t  HIL_PackRawServo(uint8_t system_id, uint8_t component_id, mavlink_servo_output_raw_t mlPwmCommands ,uint32_t time_usec)','  uint16_t  PackRawRC(uint8_t system_id, uint8_t component_id, mavlink_rc_channels_raw_t mlRC_Commands ,uint32_t time_usec)','  uint16_t  PackVFR_HUD(uint8_t system_id, uint8_t component_id, mavlink_vfr_hud_t mlVfr_hud ,uint32_t time_usec)','  char  sendQGCDebugMessage(const char * dbgMessage, char severity, unsigned char* bytesToAdd, char positionStart)','  void  TxN_Data_OverU1(uint16_t N)','  void  TxN_Data_OverU4(uint16_t N)'},1,20);s.File5=reshape({ '  float  myAtan2(float num, float denom)','  float  myPow(float x, float toTheN)','  float  mySqrt(float x)','  float  myAbs(float x)','  float  myAtan(float x)','  float  myAsin(float x)','  float  mySin(float x)','  float  myCos(float x)','  float  myTan(float x)','  float  myAcos(float x)','  float  myExp(float x)','  void  hugeDelay(void)','  void  smallDelay(void)','  void  tinyDelay(void)','  void  printToUart2(const char *fmt, ...)'},1,15);s.File6=reshape({ '  void  sendTelemetryMavlink(unsigned char* dataOut)','  void  uart2Init(void)','  void  gsRead(unsigned char* gsChunk)','  void  prepareTelemetryMavlink(unsigned char* dataOut)','  void  prepareTelemetryMavlink(unsigned char* dataOut)','  void  sendTelemetryMavlink(unsigned char* dataOut)','  void  copyBufferToDMA1(unsigned char size)','  void  send2GS(unsigned char* protData)','  uint8_t  clearWaypointsFrom(uint8_t startingWp)','  void  addMessageToSpiOut(mavlink_message_t* msg)'},1,10);s.File7={ '  void  populateParameterInterface(void)'};s.File8={ '  void  mavlinkInit(void)'};s.File9=reshape({ '  void  updatePWM(unsigned short * PWMData)','  void  updatePWMTrim(unsigned short PWMData, unsigned char channel)','  void  updateLoad(uint8_t mcuLoad)','  void  updateEuler(float* newEuler)','  void  updatePQR(float* newPQR)',' unsigned char  getHilOnOff(void)','  uint8_t  getLightsOnOff(void)','  uint8_t  getLightsDayNight(void)','  void  updateVISensor(uint16_t* data)','  void  updatePTZ(int16_t* ptz)'},1,10);s.File10=reshape({ '  void  updateRawADCData(int16_t* adcData)','  void  updateAirData(float* airData)','  void  updateLoadData(uint8_t load, uint16_t mvPower)','  void  updateAttitude(float * attitudeData)','  void  getGSLocation(float* altLatLon)','  void  updateTimeStamp(uint32_t timeSt)','  void  updatePosition(float * posData)','  void  updatePilotConsole(uint16_t * pilData)','  void  updateDiagnosticFl(float* diagFl)','  void  updateDiagnosticSh(int16_t* diagSh)','  void  updateBias(float * biasData)','  void  updateSensorData(float* sens)','  uint8_t  isFixValid(void)','  void  updateSensorDiag(float* diag)'},1,14);s.File11=reshape({ '  void  gpsInit(void)','  void  gpsParse(uint8_t* dataStream)','  void  updateStatus(uint8_t* completeMessage)','  void  updatePositionData(uint8_t* completeMessage)','  void  updateVelocityData(uint8_t* completeMessage)','  void  updateTimeData(uint8_t* completeMessage)','  void  getGpsMainData(float* data)','  uint32_t  CRC32Value(int32_t i)','  uint32_t  CalculateBlockCRC32(uint32_t ulCount, uint8_t *ucBuffer)','  uint16_t  charsToUint16(uint8_t* data)','  uint32_t  charsToUint32(uint8_t* data)','  float  charsToFloat(uint8_t* data)','  double  charsToDouble(uint8_t* data)'},1,13);s.File12=reshape({ '  void  getMidLevelCommands(float* commands)',' unsigned char  isApManual(uint16_t failsafe)','  float  getParamIdx(unsigned char idx)','  void  getRangeOfParams(uint8_t startIdx, uint8_t endIdx, float* parameters)','  float  getDynamic(void)','  void  getAttitude(float* attitude)','  void  getXYZ(float* xyz)','  void  getVned(float* xyz)','  uint8_t  getMaxWp(void)',' unsigned char  isWpFly(void)',' unsigned char  isPassthrough(void)','  void  setDiagnosticFloat(float * flValues)','  void  setDiagnosticShort(int16_t* shValues)','  void  getWP(unsigned char idx, float* WPpos)','  void  setLogFloat1(float * flValues)','  void  setLogFloat2(float * flValues)',' unsigned char  getApControlType(void)',' unsigned char  getPassValues(uint8_t* pasVals)','  void  setCurrentCommands(float airSpeed)','  void  getCurrentGPSPos(float* latLonAlt)','  void  setNavLong(float* values)','  void  setNavLat(float* values)','  void  setNavNav(float* values)','  void  getAccels(float * accels)','  void  getAccBias(float * bias)','  void  getRTB(uint8_t* rtb)','  void  getMobileLocation(float* loc)','  uint8_t  getNavMode(void)','  void  getISRLocation(float* loc)','  uint8_t  getISRCameraOption1(void)',' unsigned short  meanFilter5(unsigned short * values)','  uint8_t  justEnabled(uint8_t enableValue, uint8_t index)',' unsigned char  quickSort(unsigned short *arr, char elements)'},1,33);s.File13=reshape({ '  void  hilRead(unsigned char* hilChunk)','  void  hil_getRawRead(short * rawData)','  void  hil_getVned(float* vned)','  void  hil_getEuler(float* euler)','  void  hil_getRates(float* pqr)','  void  hil_getXYZ(float* xyz)',' unsigned int  hil_getTs(void)','  void  protDecodeHil(uint8_t* dataIn)'},1,8);s.File14=reshape({ '  void  cubeInit(void)','  void  getCubeData(short * cubeData)','  void  updateCubeData(void)','  int16_t  averageData(int16_t* theData, uint8_t count)',' unsigned short  write2Cube(unsigned short data2Send)','  short  convert14BitToShort(short wordData)','  short  convert12BitToShort(short wordData)',' unsigned char  isCube16405(void)'},1,8);s.File15=reshape({ '  void  uartMavlinkBufferInit(void)','  uint16_t  PackHeartBeat(uint8_t system_id, uint8_t component_id)','  uint16_t  PackRawServo(uint8_t system_id, uint8_t component_id, mavlink_servo_output_raw_t mlPwmCommands ,uint32_t time_usec)','  uint16_t  HIL_PackRawServo(uint8_t system_id, uint8_t component_id, mavlink_servo_output_raw_t mlPwmCommands ,uint32_t time_usec)','  uint16_t  PackRawRC(uint8_t system_id, uint8_t component_id, mavlink_rc_channels_raw_t mlRC_Commands, uint32_t time_usec)','  uint16_t  PackVFR_HUD(uint8_t system_id, uint8_t component_id, mavlink_vfr_hud_t mlVfr_hud, uint32_t time_usec)','  uint16_t  PackRawIMU(uint8_t system_id, uint8_t component_id, mavlink_raw_imu_t mlRawIMUData ,uint32_t time_usec)','  char  sendQGCDebugMessage(const char * dbgMessage, char severity, unsigned char* bytesToAdd, char positionStart)','  uint16_t  PackGpsRawInt(uint8_t system_id, uint8_t component_id, mavlink_gps_raw_int_t mlRawGpsDataInt, uint32_t time_usec)','  uint16_t  PackScaledPressure(uint8_t system_id, uint8_t component_id, mavlink_scaled_pressure_t mlAirData, uint32_t time_usec)','  uint16_t  PackSysStatus(uint8_t system_id, uint8_t component_id, mavlink_sys_status_t mlSysStatus)'},1,11);"  ORDERING=None  SampleTime=-1  MCHP_MASTERLINK=|  PinDigitalInput=[]  PinDigitalOutput=[]  PinAnalogInput=[]
      | AUAV_V3_TestSensors_/Microchip Master
      | AUAV V3 Board
      | Busy Flag on D2 (RA6)
  wires:
  PackRawServo/1 -> TX_N_Data9/1
  SYS_ID/1 -> PackRawServo/1
  Get time5/1 -> PackRawServo/4
  Get Raw Commands/1 -> PackRawServo/3
  COMP_ID/1 -> PackRawServo/2

== system AUAV_V3_TestSensors_/Barometer_Driver/Baro Altimeter/Compute Barometric Height ==
  Base Height (m) : Inport
  Base Pressure (Pa) : Inport  Port=2
  Baro (Pa) : Inport  Port=3
  Constant2 : Constant  Value=baseTemp/(-LapseRate)  OutDataTypeStr=single
  Constant3 : Constant  Value=9.350253e-2  OutDataTypeStr=single
  Constant4 : Constant  Value=-1.888933e-1  OutDataTypeStr=single
  Constant5 : Constant  Value=2.180313e-5  OutDataTypeStr=single
  Divide : Product  Inputs=*/  OutDataTypeStr=single
  Divide{1..4} (4 alike) : Product  OutDataTypeStr=single
  Length Conversion : aerolibconvert2/Length Conversion  IU=ft  OU=m
  Sum1 : Sum  Inputs=|++  OutDataTypeStr=single
  Sum2 : Sum  Inputs=|+-  OutDataTypeStr=single
  Sum3 : Sum  Inputs=3  OutDataTypeStr=single
  "Altitude, m" : Outport
  wires:
  Baro (Pa)/1 -> Sum2/1
  Base Height (m)/1 -> Sum1/2
  Base Pressure (Pa)/1 -> Sum2/2, Divide/2
  Divide/1 -> Divide4/2, Divide4/1, Divide2/1  "x"
  Divide4/1 -> Divide1/1  "x^2"
  Constant3/1 -> Divide1/2
  Constant4/1 -> Divide2/2
  Divide1/1 -> Sum3/1
  Divide2/1 -> Sum3/2
  Constant5/1 -> Sum3/3
  Sum3/1 -> Divide3/1
  Constant2/1 -> Divide3/2
  Divide3/1 -> Length Conversion/1
  Sum1/1 -> "Altitude, m"/1
  Sum2/1 -> Divide/1
  Length Conversion/1 -> Sum1/1

== system AUAV_V3_TestSensors_/Barometer_Driver/Baro Altimeter/Enabled Subsystem ==
  In1 : Inport
  Enable : EnablePort
  Out1 : Outport  InitialOutput=baseHeight
  wires:
  In1/1 -> Out1/1

== system AUAV_V3_TestSensors_/Barometer_Driver/Baro Altimeter/Initial Baro Bias ==
  Baro (Pa) : Inport
  Enable : EnablePort
  Data Type Conversion : DataTypeConversion  OutDataTypeStr=double
  Data Type Conversion1 : DataTypeConversion  OutDataTypeStr=single
  Low Pass8 : Subsystem  mask(DiscretizedZeroPole){Zeros=[], Poles=[-3], Gain=3, AbsTol=auto, SampleTime=.01, method=tustin, Wc=1}
      mask prompts: Zeros "Zeros (enter in s-main:)"; Poles "Poles (enter in s-domain:)"; Gain "Gain (enter in s-domain:)"; AbsTol "Absolute tolerance:"; SampleTime "Sample time:"; Wc "Critical Frequency (Hz):"
      mask help: Continuous mask uses c2d to transform parameters onto the Discrete Zero-Pole block inside.
      mask init:
      | st=SampleTime;
      | if length(st)>1
      |     st=SampleTime(1);
      | end
      | if(st>0)
      |     [zerosd,polesd,gaind] = sldiscutil('disczpk', {st,method,Wc,Zeros,Poles,Gain});
      | end	
      | s = get_param(gcb,'maskvalues');
      | zeross = s{1};
      | poless = s{2};
      | gainss = s{3};
      | %zerosc = eval(zeross);
      | %polesc = eval(poless);
      | %gainsc = eval(gainss);
      | sldiscutil('initzpkmask', st);
      | if(st==0)
      | set_param([gcb '/Zero Pole'], 'AbsoluteTolerance', AbsTol);
      | end
      mask TypeOptions method: zoh | foh | tustin | prewarp | matched
      mask Callback method: hidecrit
      mask Display:
      | droots(zeross,poless,gainss)
      | text( 0.5, 1.0, method, 'verticalAlignment','top')
  "[80k - 120k]" : Saturate  UpperLimit=120000  LowerLimit=80000
  Baro (Gnd) : Outport
  wires:
  "[80k - 120k]"/1 -> Baro (Gnd)/1
  Data Type Conversion1/1 -> "[80k - 120k]"/1
  Data Type Conversion/1 -> Low Pass8/1(In1)
  Low Pass8/1(Out1) -> Data Type Conversion1/1
  Baro (Pa)/1 -> Data Type Conversion/1
